simulink model "modeloInfeccion4"  (R2021a)
settings: Solver=VariableStepAuto  StartTime=0.0  StopTime=1000  RelTol=1e-3
settings Model: Creator=jmata  LastModifiedBy=jmata

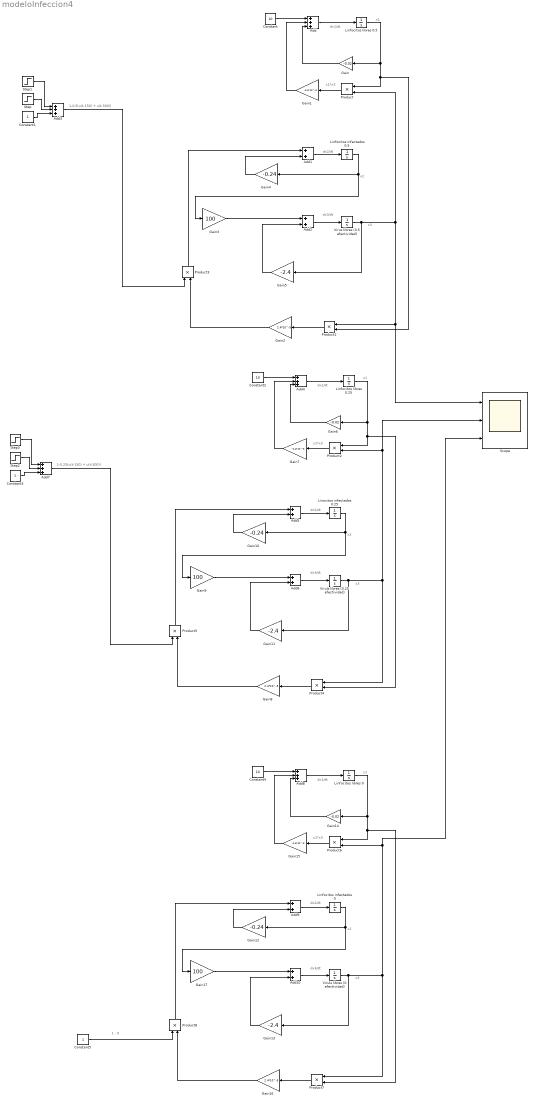
== system modeloInfeccion4 ==
  note: 1 - 0
  note: 1-0.5(u(t-150) + u(t-500))
  note: dx3/dt
  note: x3
  note: x2
  note: x1*x3
  note: x1
  note: dx1/dt
  note: dx2/dt
  note: 1-0.25(u(t-150) + u(t-500))
  note: dx3/dt
  note: x3
  note: x2
  note: x1*x3
  note: x1
  note: dx1/dt
  note: dx2/dt
  note: dx3/dt
  note: x3
  note: x2
  note: x1*x3
  note: x1
  note: dx1/dt
  note: dx2/dt
  Add{,3..4,7..8} (5 alike) : Sum  Inputs=+++
  Add{1..2,5..6,9..10} (6 alike) : Sum
  Constant : Constant  Value=10
  Constant1 : Constant
  Constant2 : Constant  Value=10
  Constant3 : Constant
  Constant4 : Constant  Value=10
  Constant5 : Constant
  Gain : Gain  Gain=-0.02
  Gain1 : Gain  Gain=-2.4*10^-5
  Gain10 : Gain  Gain=-0.24
  Gain11 : Gain  Gain=-2.4
  Gain12 : Gain  Gain=-0.24
  Gain13 : Gain  Gain=-2.4
  Gain14 : Gain  Gain=-0.02
  Gain15 : Gain  Gain=-2.4*10^-5
  Gain16 : Gain  Gain=2.4*10^-5
  Gain17 : Gain  Gain=100
  Gain2 : Gain  Gain=2.4*10^-5
  Gain3 : Gain  Gain=100
  Gain4 : Gain  Gain=-0.24
  Gain5 : Gain  Gain=-2.4
  Gain6 : Gain  Gain=-0.02
  Gain7 : Gain  Gain=-2.4*10^-5
  Gain8 : Gain  Gain=2.4*10^-5
  Gain9 : Gain  Gain=100
  Linfocitos infectados 0 : Integrator
  Linfocitos infectados 0.5 : Integrator
  Linfocitos libres 0 : Integrator  InitialCondition=500
  Linfocitos libres 0.25 : Integrator  InitialCondition=500
  Linfocitos libres 0.5 : Integrator  InitialCondition=500
  Linocitos infectados 0.25 : Integrator
  Product{,1..8} (9 alike) : Product
  Scope : Scope  NumInputPorts=3
  Step : Step  After=-0.5  SampleTime=150
  Step1 : Step  After=+0.5  SampleTime=500
  Step2 : Step  After=-0.25  SampleTime=150
  Step3 : Step  After=+0.25  SampleTime=500
  Viruls libres (0 efectividad) : Integrator  InitialCondition=1
  Viruls libres (0.25 efectividad) : Integrator  InitialCondition=1
  Virus libres (0.5 efectividad) : Integrator  InitialCondition=1
  wires:
  Gain2/1 -> Product3/2
  Gain3/1 -> Add2/1
  Constant1/1 -> Add3/3
  Product1/1 -> Gain2/1
  Product/1 -> Gain1/1
  Step/1 -> Add3/2
  Virus libres (0.5 efectividad)/1 -> Gain5/1, Scope/1, Product1/1, Product/2
  Product3/1 -> Add1/1
  Constant/1 -> Add/1
  Add1/1 -> Linfocitos infectados 0.5/1
  Gain4/1 -> Add1/2
  Linfocitos libres 0.5/1 -> Product/1, Product1/2, Gain/1
  Gain1/1 -> Add/2
  Add2/1 -> Virus libres (0.5 efectividad)/1
  Linfocitos infectados 0.5/1 -> Gain3/1, Gain4/1
  Gain/1 -> Add/3
  Add/1 -> Linfocitos libres 0.5/1
  Gain5/1 -> Add2/2
  Add3/1 -> Product3/1
  Step1/1 -> Add3/1
  Step3/1 -> Add7/1
  Add7/1 -> Product5/1
  Gain11/1 -> Add6/2
  Add4/1 -> Linfocitos libres 0.25/1
  Gain6/1 -> Add4/3
  Linocitos infectados 0.25/1 -> Gain10/1, Gain9/1
  Add6/1 -> Viruls libres (0.25 efectividad)/1
  Gain7/1 -> Add4/2
  Linfocitos libres 0.25/1 -> Gain6/1, Product4/2, Product2/1
  Gain10/1 -> Add5/2
  Add5/1 -> Linocitos infectados 0.25/1
  Constant2/1 -> Add4/1
  Product5/1 -> Add5/1
  Viruls libres (0.25 efectividad)/1 -> Scope/2, Product2/2, Product4/1, Gain11/1
  Step2/1 -> Add7/2
  Product2/1 -> Gain7/1
  Product4/1 -> Gain8/1
  Constant3/1 -> Add7/3
  Gain9/1 -> Add6/1
  Gain8/1 -> Product5/2
  Gain16/1 -> Product8/2
  Gain17/1 -> Add10/1
  Product7/1 -> Gain16/1
  Product6/1 -> Gain15/1
  Product8/1 -> Add9/1
  Constant4/1 -> Add8/1
  Add9/1 -> Linfocitos infectados 0/1
  Gain12/1 -> Add9/2
  Linfocitos libres 0/1 -> Product6/1, Product7/2, Gain14/1
  Gain15/1 -> Add8/2
  Add10/1 -> Viruls libres (0 efectividad)/1
  Linfocitos infectados 0/1 -> Gain17/1, Gain12/1
  Gain14/1 -> Add8/3
  Add8/1 -> Linfocitos libres 0/1
  Gain13/1 -> Add10/2
  Constant5/1 -> Product8/1
  Viruls libres (0 efectividad)/1 -> Gain13/1, Product7/1, Scope/3, Product6/2
